simulink model "Subsystem"  (R2024b)
settings: Solver=VariableStepAuto  StartTime=0.0  StopTime=10.0  RelTol=1e-3
settings Model: DataDictionary=Data.sldd  Creator=toma  LastModifiedBy=toma
settings DataIOCC: SaveOutput=off  SaveTime=off
settings ConfigComp: CovBoundaryAbsTol=1.0e-5

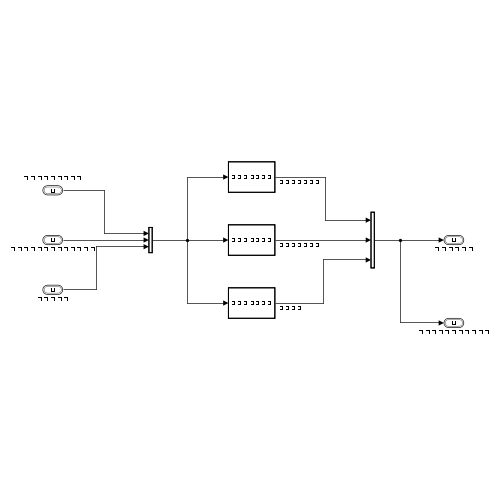
[thumbnail: Simulink's stored preview of the top-level diagram]
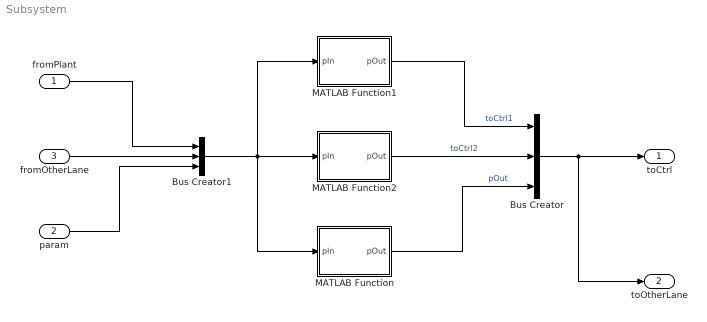
== system Subsystem ==
  fromPlant : Inport  OutDataTypeStr=Bus: PlantOut  PortDimensions=1  BusOutputAsStruct=on
  param : Inport  Port=2  OutDataTypeStr=Bus: ExtParams  PortDimensions=1  BusOutputAsStruct=on
  fromOtherLane : Inport  Port=3  OutDataTypeStr=Bus: toCtrl  BusOutputAsStruct=on
  Bus Creator : BusCreator  Inputs=3  OutDataTypeStr=Bus: toCtrl  NonVirtualBus=on
      settings: InheritFromInputs=off
  Bus Creator1 : BusCreator  Inputs=3  OutDataTypeStr=Bus: topLevelIn  NonVirtualBus=on
      settings: InheritFromInputs=off
  MATLAB Function : MATLAB Function  TreatAsAtomicUnit=on
  MATLAB Function1 : MATLAB Function  TreatAsAtomicUnit=on
  MATLAB Function2 : MATLAB Function  TreatAsAtomicUnit=on
  toCtrl : Outport  OutDataTypeStr=Bus: toCtrl  PortDimensions=1
  toOtherLane : Outport  Port=2  OutDataTypeStr=Bus: toCtrl
  wires:
  MATLAB Function1/1(pOut) -> Bus Creator/1  "toCtrl1"
  MATLAB Function/1(pOut) -> Bus Creator/3  "pOut"
  param/1 -> Bus Creator1/3
  Bus Creator/1 -> toOtherLane/1, toCtrl/1
  MATLAB Function2/1(pOut) -> Bus Creator/2  "toCtrl2"
  fromPlant/1 -> Bus Creator1/1
  fromOtherLane/1 -> Bus Creator1/2
  Bus Creator1/1 -> MATLAB Function/1(pIn), MATLAB Function1/1(pIn), MATLAB Function2/1(pIn)

== matlab function Subsystem/MATLAB Function ==
  data: pIn input Bus: topLevelIn; pOut output Bus: Params
function pOut = fcn(pIn)

pOut.p = pIn.param.p_ext;
pOut.p1 = pIn.param.p1_ext;
pOut.p2 = pIn.param.p2_ext;

end

== matlab function Subsystem/MATLAB Function2 ==
  data: pIn input Bus: topLevelIn; pOut output Bus: InBus
function pOut = fcn(pIn)

pOut = mapToPlant(pIn);

end

== matlab function Subsystem/MATLAB Function1 ==
  data: pIn input Bus: topLevelIn; pOut output Bus: InBus
function pOut = fcn(pIn)

pOut = mapToPlant(pIn);

end
